simulink model "QuadSim"  (R2016a)
settings: Solver=FixedStepAuto  StartTime=0.0  StopTime=10  FixedStep=0.001  RelTol=1e-3
InitFcn:
  | Parameters
StartFcn:
  | Parameters
values from neighbouring files (symbols this model uses):
  b = 4.5*10^-4    (= 0.00045)    [Parameters.m]
  d = 1.8*10^-5    (= 1.8e-05)    [Parameters.m]
  g = 9.81    [Parameters.m]
  I = [7.06 0 0;0 7.06 0; 0 0 7.865]*10^-3    [Parameters.m]
  IC_orient = [0;0;0]    [Parameters.m]
  IC_pos = [0;0;0]    [Parameters.m]
  IC_rot_vel = [0;0;0]    [Parameters.m]
  IC_trans_vel = [0;0;0]    [Parameters.m]
  J_TP = 14.2*10^-4    (= 0.00142)    [Parameters.m]
  l = 8.25    [Parameters.m]
  m = 1.8    [Parameters.m]
settings Model: Creator=Chris  LastModifiedBy=Chris

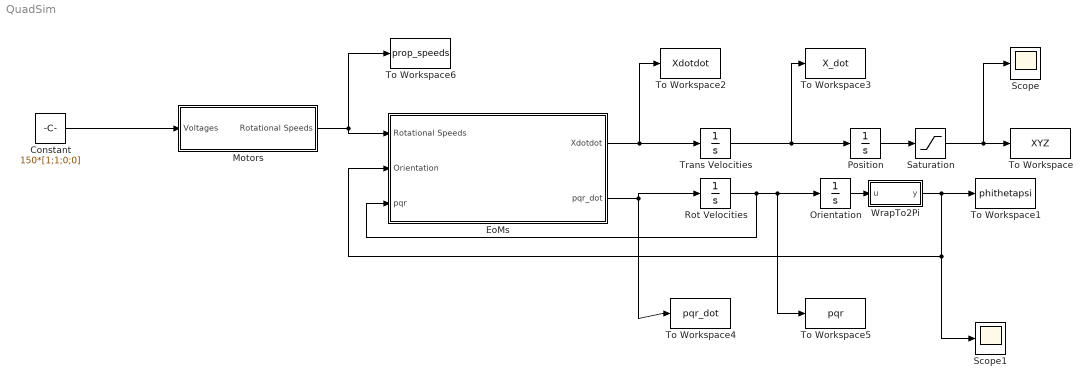
== system QuadSim ==
  Constant : Constant  Value=150*[1;1;0;0]
  EoMs : Subsystem
  Motors : Subsystem
  Orientation : Integrator  InitialCondition=[IC_orient]
  Position : Integrator  InitialCondition=[IC_pos]
  Rot Velocities : Integrator  InitialCondition=[IC_rot_vel]
  Saturation : Saturate  UpperLimit=1e99  LowerLimit=0
  Scope : Scope
  Scope1 : Scope
  To Workspace : ToWorkspace  VariableName=XYZ  SampleTime=-1
  To Workspace1 : ToWorkspace  VariableName=phithetapsi  SampleTime=-1
  To Workspace2 : ToWorkspace  VariableName=Xdotdot  SampleTime=-1
  To Workspace3 : ToWorkspace  VariableName=X_dot  SampleTime=-1
  To Workspace4 : ToWorkspace  VariableName=pqr_dot  SampleTime=-1
  To Workspace5 : ToWorkspace  VariableName=pqr  SampleTime=-1
  To Workspace6 : ToWorkspace  VariableName=prop_speeds  SampleTime=-1
  Trans Velocities : Integrator  InitialCondition=[IC_trans_vel]
  WrapTo2Pi : MATLAB Function  TreatAsAtomicUnit=on
  wires:
  Motors/1(Rotational Speeds) -> To Workspace6/1, EoMs/1(Rotational Speeds)
  EoMs/1(Xdotdot) -> To Workspace2/1, Trans Velocities/1
  Trans Velocities/1 -> To Workspace3/1, Position/1
  EoMs/2(pqr_dot) -> To Workspace4/1, Rot Velocities/1
  Rot Velocities/1 -> Orientation/1, To Workspace5/1, EoMs/3(pqr)
  Orientation/1 -> WrapTo2Pi/1(u)
  Position/1 -> Saturation/1
  Constant/1 -> Motors/1(Voltages)
  WrapTo2Pi/1(y) -> EoMs/2(Orientation), Scope1/1, To Workspace1/1
  Saturation/1 -> Scope/1, To Workspace/1

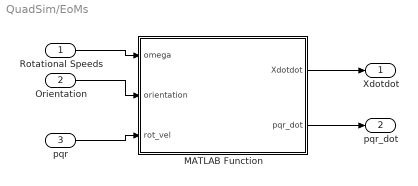
== system QuadSim/EoMs ==
  Rotational Speeds : Inport
  Orientation : Inport  Port=2
  pqr : Inport  Port=3
  MATLAB Function : MATLAB Function  TreatAsAtomicUnit=on
  Xdotdot : Outport
  pqr_dot : Outport  Port=2
  wires:
  MATLAB Function/1(Xdotdot) -> Xdotdot/1
  Rotational Speeds/1 -> MATLAB Function/1(omega)
  Orientation/1 -> MATLAB Function/2(orientation)
  pqr/1 -> MATLAB Function/3(rot_vel)
  MATLAB Function/2(pqr_dot) -> pqr_dot/1

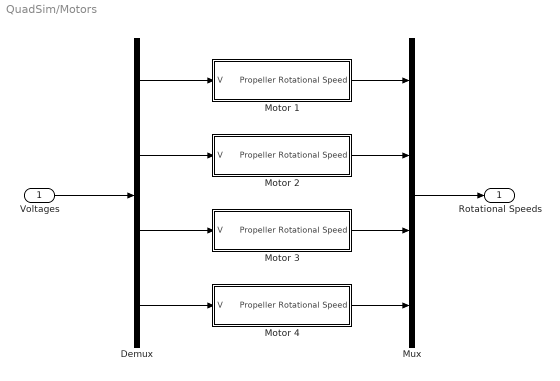
== system QuadSim/Motors ==
  Voltages : Inport
  Demux : Demux
  "Motor 1 " : Subsystem
  Motor 2 : Subsystem
  Motor 3 : Subsystem
  "Motor 4 " : Subsystem
  Mux : Mux
  Rotational Speeds : Outport
  wires:
  Voltages/1 -> Demux/1
  Mux/1 -> Rotational Speeds/1
  "Motor 1 "/1(Propeller Rotational Speed) -> Mux/1
  Motor 2/1(Propeller Rotational Speed) -> Mux/2
  Motor 3/1(Propeller Rotational Speed) -> Mux/3
  "Motor 4 "/1(Propeller Rotational Speed) -> Mux/4
  Demux/4 -> "Motor 4 "/1(V)
  Demux/3 -> Motor 3/1(V)
  Demux/2 -> Motor 2/1(V)
  Demux/1 -> "Motor 1 "/1(V)

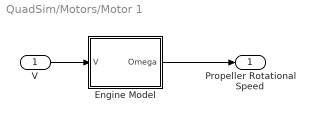
== system QuadSim/Motors/Motor 1  ==
  V : Inport
  Engine Model : MATLAB Function  TreatAsAtomicUnit=on
  Propeller Rotational Speed : Outport
  wires:
  Engine Model/1(Omega) -> Propeller Rotational Speed/1
  V/1 -> Engine Model/1(V)

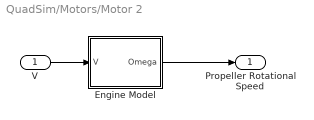
== system QuadSim/Motors/Motor 2 ==
  V : Inport
  Engine Model : MATLAB Function  TreatAsAtomicUnit=on
  Propeller Rotational Speed : Outport
  wires:
  Engine Model/1(Omega) -> Propeller Rotational Speed/1
  V/1 -> Engine Model/1(V)

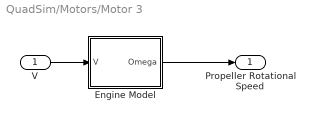
== system QuadSim/Motors/Motor 3 ==
  V : Inport
  Engine Model : MATLAB Function  TreatAsAtomicUnit=on
  Propeller Rotational Speed : Outport
  wires:
  Engine Model/1(Omega) -> Propeller Rotational Speed/1
  V/1 -> Engine Model/1(V)

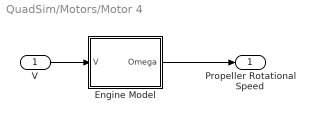
== system QuadSim/Motors/Motor 4  ==
  V : Inport
  Engine Model : MATLAB Function  TreatAsAtomicUnit=on
  Propeller Rotational Speed : Outport
  wires:
  Engine Model/1(Omega) -> Propeller Rotational Speed/1
  V/1 -> Engine Model/1(V)

== matlab function QuadSim/Motors/Motor 2/Engine Model ==
  data: V input; Omega output
function Omega  = fcn(V)
%#codegen
Omega = V;

== matlab function QuadSim/Motors/Motor 1 /Engine Model ==
  data: V input; Omega output
function Omega  = fcn(V)
%#codegen
Omega = V;

== matlab function QuadSim/Motors/Motor 4 /Engine Model ==
  data: V input; Omega output
function Omega  = fcn(V)
%#codegen
Omega = V;

== matlab function QuadSim/Motors/Motor 3/Engine Model ==
  data: V input; Omega output
function Omega  = fcn(V)
%#codegen
Omega = V;

== matlab function QuadSim/EoMs/MATLAB Function ==
  data: omega input; Xdotdot output; orientation input; rot_vel input; g parameter; m parameter; I parameter; J_TP parameter; pqr_dot output; b parameter; d parameter; l parameter
function [Xdotdot, pqr_dot] = fcn(omega,orientation,rot_vel,g, m, I, J_TP, b, d, l)
%#codegen
phi = orientation(1);
theta = orientation(2);
psi = orientation(3);

R=rotMat(psi,theta,phi);

Ixx = I(1,1);
Iyy = I(2,2);
Izz = I(3,3);

% u = trans_vel(1);
% v = trans_vel(2);
% w = trans_vel(3);

p = rot_vel(1);
q = rot_vel(2);
r = rot_vel(3);

TB = [0;0;b*sum(omega.^2)];
TauB = [l*b*(omega(1)^2-omega(3)^2);...
           l*b*(omega(2)^2-omega(4)^2);...
           d*(omega(1)^2-omega(2)^2+omega(3)^2-omega(4)^2)];

pqr_dot = zeros(3,1);
Xdotdot = [0;0;-g] + R*TB/m;
pqr_dot(1) = TauB(1)*Ixx^-1-(Iyy-Izz)/Ixx*q*r;
pqr_dot(2) = TauB(2)*Iyy^-1-(Izz-Ixx)/Iyy*p*r;
pqr_dot(3) = TauB(3)*Izz^-1-(Ixx-Iyy)/Izz*p*q;

% U1 = b*(omega(1)^2+omega(2)^2+omega(3)^2+omega(4)^2);
% U2 = l*b*(-omega(1)^2-omega(2)^2+omega(3)^2+omega(4)^2);
% U3 = l*b*(omega(1)^2-omega(2)^2-omega(3)^2+omega(4)^2);
% U4 = d*(-omega(1)^2+omega(2)^2-omega(3)^2+omega(4)^2);
% Omega = b*(omega(1)^2-omega(2)^2+omega(3)^2-omega(4)^2);
% 
% u_dot = (v*r-w*q) + g*sin(theta);
% v_dot = (w*p-u*r) - g*cos(theta)*sin(phi);
% w_dot = (u*q-v*p) - g*cos(theta)*sin(theta)+U1/m;
% 
% p_dot = (Iyy-Izz)/Izz*q*r - J_TP/Ixx*q*Omega + U2/Ixx;
% q_dot = (Izz-Ixx)/Iyy*p*r - J_TP/Iyy*p*Omega + U3/Iyy;
% r_dot = (Ixx-Iyy)/Izz*p*q - J_TP/Izz + U4/Izz;
% 
% uvw_dot = [u_dot;v_dot;w_dot];
% pqr_dot = [p_dot;q_dot;r_dot];

== matlab function QuadSim/WrapTo2Pi ==
  data: u input; y output
function y = fcn(u)
%#codegen
y = [mod(u(1),2*pi);mod(u(2),2*pi);mod(u(3),2*pi)];
